simulink model "sigma_delta_1er_ordre_TP"  (Simulink 6.2)
settings: Solver=ode3  StartTime=0.0  StopTime=1-ts  FixedStep=ts  RelTol=1e-3
values from neighbouring files (symbols this model uses):
  fck = 1000000    [main_sigma_delta.m]
  noise_laplace = 10^-10    (= 1e-10)    [main_sigma_delta.m]
  tau = 1/(2*pi*fc)    (= 0.0159154943092)    [main_sigma_delta.m]
  ts = 0.000001    (= 1e-06)    [main_sigma_delta.m]
libraries: simulink x1
settings Model: LastModifiedBy=Mailly
settings DebuggingCC: SolverPrmCheckMsg=warning

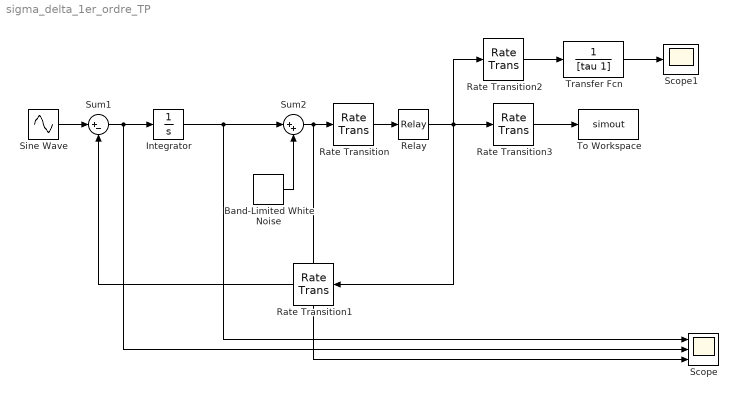
== system sigma_delta_1er_ordre_TP ==
  Band-Limited White Noise : simulink/Sources/Band-Limited White Noise  Cov=[noise_laplace]  Ts=ts  seed=[23341]
  Integrator : Integrator
  Rate Transition : RateTransition
  Rate Transition1 : RateTransition  Orientation=left
  Rate Transition2 : RateTransition
  Rate Transition3 : RateTransition
  Relay : Relay  OnSwitchValue=0  OffSwitchValue=0  OffOutputValue=-1  SampleTime=1/fck
  Scope : Scope  NumInputPorts=3
      settings: YMin=-0.0002~-1~-0.00025  YMax=0.0002~1~0.00025
  Scope1 : Scope
      settings: YMin=-1  YMax=1
  Sine Wave : Sin  Amplitude=0.5  Frequency=2*pi*250  SampleTime=ts
  Sum1 : Sum  Inputs=|+-
  Sum2 : Sum  Inputs=|++
  To Workspace : ToWorkspace  VariableName=simout  SampleTime=ts  SaveFormat=Array
      settings: MaxDataPoints=fck
  Transfer Fcn : TransferFcn  Denominator=[tau 1]
  wires:
  Sine Wave/1 -> Sum1/1
  Sum1/1 -> Scope/2, Integrator/1
  Relay/1 -> Rate Transition1/1, Rate Transition2/1, Rate Transition3/1
  Rate Transition1/1 -> Sum1/2
  Band-Limited White Noise/1 -> Sum2/2
  Sum2/1 -> Rate Transition/1, Scope/3
  Rate Transition/1 -> Relay/1
  Transfer Fcn/1 -> Scope1/1
  Rate Transition2/1 -> Transfer Fcn/1
  Integrator/1 -> Sum2/1, Scope/1
  Rate Transition3/1 -> To Workspace/1
